simulink model "nonlin_quadro_orig"  (R2020b)
settings: Solver=VariableStepAuto  StartTime=0.0  StopTime=10.0  RelTol=1e-3
values from neighbouring files (symbols this model uses):
  b = 26.5e-6    (= 2.65e-05)    [quadro_new_ast_test.m]
  d = 0.6e-6    (= 6e-07)    [quadro_new_ast_test.m]
  g = 9.80665    [quadro_new_ast_test.m]
  Ixx = 0.1    [quadro_new_ast_test.m]
  Iyy = 0.1    [quadro_new_ast_test.m]
  Izz = 0.1    [quadro_new_ast_test.m]
  JTP = 0.005    [quadro_new_ast_test.m]
  l = 0.175    [quadro_new_ast_test.m]
  m = 1    [quadro_new_ast_test.m]
settings Model: Creator=Наташа  LastModifiedBy=Наташа

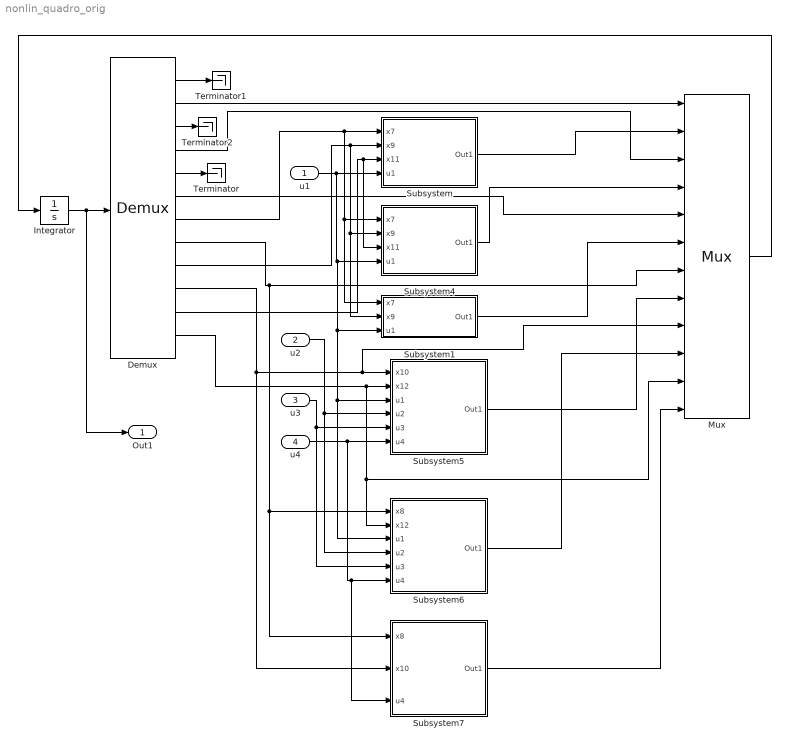
== system nonlin_quadro_orig ==
  u1 : Inport
  u2 : Inport  Port=2
  u3 : Inport  Port=3
  u4 : Inport  Port=4
  Demux : Demux  Outputs=12
  Integrator : Integrator
  Mux : Mux  Inputs=12
  Subsystem : Subsystem
  Subsystem1 : Subsystem
  Subsystem4 : Subsystem
  Subsystem5 : Subsystem
  Subsystem6 : Subsystem
  Subsystem7 : Subsystem
  Terminator : Terminator
  Terminator1 : Terminator
  Terminator2 : Terminator
  Out1 : Outport
  wires:
  Subsystem4/1(Out1) -> Mux/4
  Demux/4 -> Mux/3
  Demux/1 -> Terminator1/1
  Demux/3 -> Terminator2/1
  Demux/5 -> Terminator/1
  Subsystem6/1(Out1) -> Mux/10
  Subsystem5/1(Out1) -> Mux/8
  Demux/7 -> Subsystem1/1(x7), Subsystem4/1(x7), Subsystem/1(x7)
  u3/1 -> Subsystem6/5(u3), Subsystem5/5(u3)
  u4/1 -> Subsystem7/3(u4), Subsystem6/6(u4), Subsystem5/6(u4)
  Subsystem1/1(Out1) -> Mux/6
  u2/1 -> Subsystem6/4(u2), Subsystem5/4(u2)
  Demux/8 -> Subsystem7/1(x8), Subsystem6/1(x8), Mux/7
  Demux/9 -> Subsystem/2(x9), Subsystem1/2(x9), Subsystem4/2(x9)
  Mux/1 -> Integrator/1
  Demux/12 -> Mux/11, Subsystem6/2(x12), Subsystem5/2(x12)
  Demux/10 -> Subsystem7/2(x10), Mux/9, Subsystem5/1(x10)
  u1/1 -> Subsystem6/3(u1), Subsystem5/3(u1), Subsystem1/3(u1), Subsystem4/4(u1), Subsystem/4(u1)
  Demux/6 -> Mux/5
  Subsystem/1(Out1) -> Mux/2
  Demux/11 -> Subsystem4/3(x11), Subsystem/3(x11)
  Integrator/1 -> Out1/1, Demux/1
  Demux/2 -> Mux/1
  Subsystem7/1(Out1) -> Mux/12

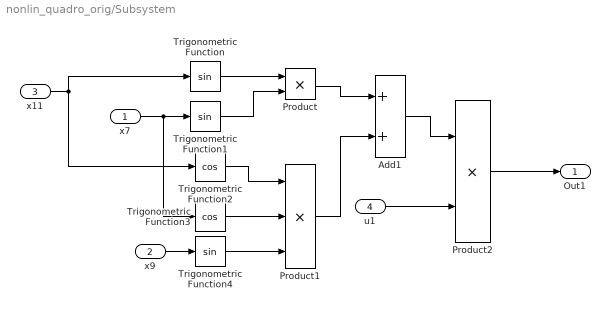
== system nonlin_quadro_orig/Subsystem ==
  x7 : Inport
  x9 : Inport  Port=2
  x11 : Inport  Port=3
  u1 : Inport  Port=4
  Add1 : Sum
  Product : Product
  Product1 : Product  Inputs=3
  Product2 : Product
  Trigonometric Function : Trigonometry
  Trigonometric Function1 : Trigonometry
  Trigonometric Function2 : Trigonometry  Operator=cos
  Trigonometric Function3 : Trigonometry  Operator=cos
  Trigonometric Function4 : Trigonometry
  Out1 : Outport
  wires:
  x11/1 -> Trigonometric Function/1, Trigonometric Function2/1
  Trigonometric Function/1 -> Product/1
  Trigonometric Function1/1 -> Product/2
  x7/1 -> Trigonometric Function3/1, Trigonometric Function1/1
  Product/1 -> Add1/1
  x9/1 -> Trigonometric Function4/1
  Trigonometric Function2/1 -> Product1/1
  Trigonometric Function3/1 -> Product1/2
  Trigonometric Function4/1 -> Product1/3
  Product1/1 -> Add1/2
  Add1/1 -> Product2/1
  u1/1 -> Product2/2
  Product2/1 -> Out1/1

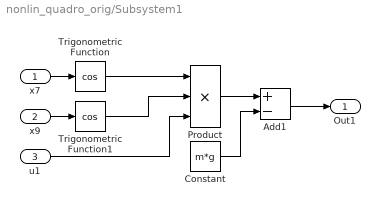
== system nonlin_quadro_orig/Subsystem1 ==
  x7 : Inport
  x9 : Inport  Port=2
  u1 : Inport  Port=3
  Add1 : Sum  Inputs=+-
  Constant : Constant  Value=m*g
  Product : Product  Inputs=3
  Trigonometric Function : Trigonometry  Operator=cos
  Trigonometric Function1 : Trigonometry  Operator=cos
  Out1 : Outport
  wires:
  x7/1 -> Trigonometric Function/1
  x9/1 -> Trigonometric Function1/1
  Trigonometric Function/1 -> Product/1
  Trigonometric Function1/1 -> Product/2
  u1/1 -> Product/3
  Product/1 -> Add1/1
  Constant/1 -> Add1/2
  Add1/1 -> Out1/1

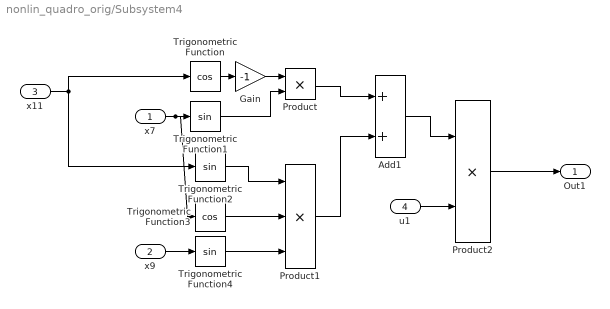
== system nonlin_quadro_orig/Subsystem4 ==
  x7 : Inport
  x9 : Inport  Port=2
  x11 : Inport  Port=3
  u1 : Inport  Port=4
  Add1 : Sum
  Gain : Gain  Gain=-1
  Product : Product
  Product1 : Product  Inputs=3
  Product2 : Product
  Trigonometric Function : Trigonometry  Operator=cos
  Trigonometric Function1 : Trigonometry
  Trigonometric Function2 : Trigonometry
  Trigonometric Function3 : Trigonometry  Operator=cos
  Trigonometric Function4 : Trigonometry
  Out1 : Outport
  wires:
  Product2/1 -> Out1/1
  u1/1 -> Product2/2
  Add1/1 -> Product2/1
  Product1/1 -> Add1/2
  Trigonometric Function4/1 -> Product1/3
  Trigonometric Function3/1 -> Product1/2
  Trigonometric Function2/1 -> Product1/1
  x9/1 -> Trigonometric Function4/1
  Product/1 -> Add1/1
  x7/1 -> Trigonometric Function3/1, Trigonometric Function1/1
  Trigonometric Function1/1 -> Product/2
  x11/1 -> Trigonometric Function2/1, Trigonometric Function/1
  Trigonometric Function/1 -> Gain/1
  Gain/1 -> Product/1

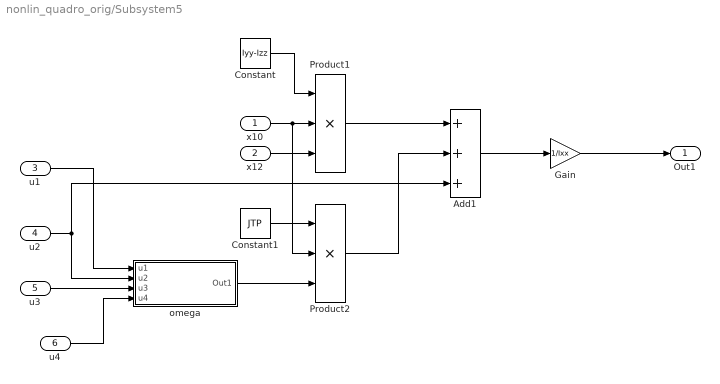
== system nonlin_quadro_orig/Subsystem5 ==
  x10 : Inport
  x12 : Inport  Port=2
  u1 : Inport  Port=3
  u2 : Inport  Port=4
  u3 : Inport  Port=5
  u4 : Inport  Port=6
  Add1 : Sum  Inputs=+++
  Constant : Constant  Value=Iyy-Izz
  Constant1 : Constant  Value=JTP
  Gain : Gain  Gain=1/Ixx
  Product1 : Product  Inputs=3
  Product2 : Product  Inputs=3
  omega : Subsystem
  Out1 : Outport
  wires:
  Constant/1 -> Product1/1
  x10/1 -> Product2/2, Product1/2
  x12/1 -> Product1/3
  Constant1/1 -> Product2/1
  omega/1(Out1) -> Product2/3
  u1/1 -> omega/1(u1)
  u2/1 -> omega/2(u2), Add1/3
  u3/1 -> omega/3(u3)
  u4/1 -> omega/4(u4)
  Product1/1 -> Add1/1
  Product2/1 -> Add1/2
  Add1/1 -> Gain/1
  Gain/1 -> Out1/1

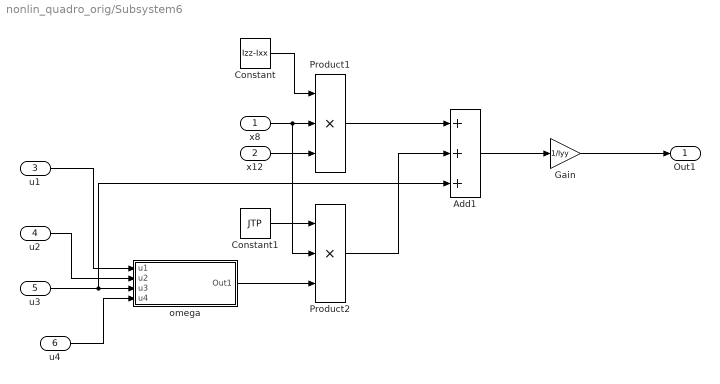
== system nonlin_quadro_orig/Subsystem6 ==
  x8 : Inport
  x12 : Inport  Port=2
  u1 : Inport  Port=3
  u2 : Inport  Port=4
  u3 : Inport  Port=5
  u4 : Inport  Port=6
  Add1 : Sum  Inputs=+++
  Constant : Constant  Value=Izz-Ixx
  Constant1 : Constant  Value=JTP
  Gain : Gain  Gain=1/Iyy
  Product1 : Product  Inputs=3
  Product2 : Product  Inputs=3
  omega : Subsystem
  Out1 : Outport
  wires:
  Gain/1 -> Out1/1
  Add1/1 -> Gain/1
  Product2/1 -> Add1/2
  Product1/1 -> Add1/1
  u4/1 -> omega/4(u4)
  u3/1 -> Add1/3, omega/3(u3)
  u2/1 -> omega/2(u2)
  u1/1 -> omega/1(u1)
  omega/1(Out1) -> Product2/3
  Constant1/1 -> Product2/1
  x12/1 -> Product1/3
  x8/1 -> Product1/2, Product2/2
  Constant/1 -> Product1/1

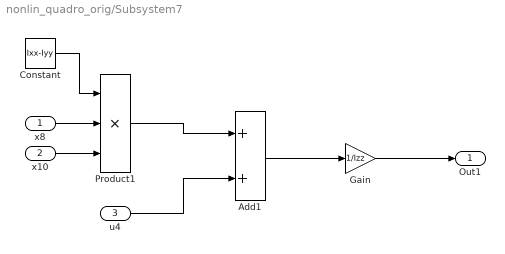
== system nonlin_quadro_orig/Subsystem7 ==
  x8 : Inport
  x10 : Inport  Port=2
  u4 : Inport  Port=3
  Add1 : Sum
  Constant : Constant  Value=Ixx-Iyy
  Gain : Gain  Gain=1/Izz
  Product1 : Product  Inputs=3
  Out1 : Outport
  wires:
  Constant/1 -> Product1/1
  x8/1 -> Product1/2
  x10/1 -> Product1/3
  Product1/1 -> Add1/1
  Add1/1 -> Gain/1
  Gain/1 -> Out1/1
  u4/1 -> Add1/2

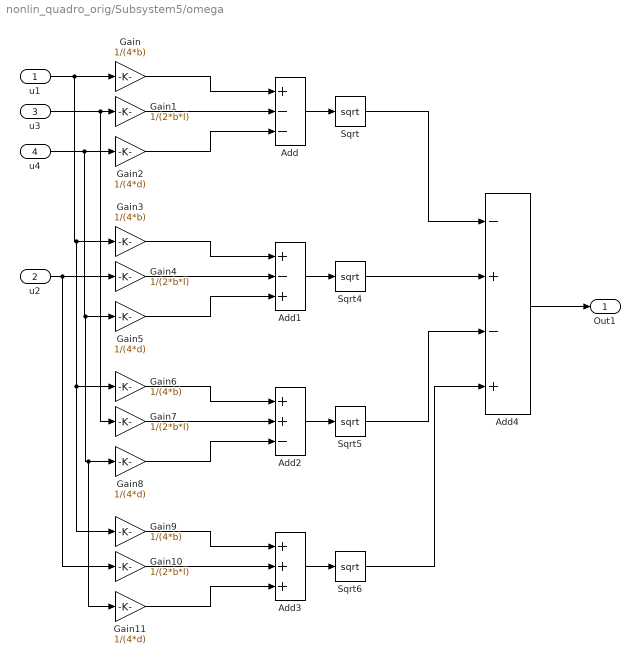
== system nonlin_quadro_orig/Subsystem5/omega ==
  u1 : Inport
  u2 : Inport  Port=2
  u3 : Inport  Port=3
  u4 : Inport  Port=4
  Add : Sum  Inputs=+--
  Add1 : Sum  Inputs=+-+
  Add2 : Sum  Inputs=++-
  Add3 : Sum  Inputs=+++
  Add4 : Sum  Inputs=-+-+
  Gain{,3,6,9} (4 alike) : Gain  Gain=1/(4*b)
  Gain{1,4,7,10} (4 alike) : Gain  Gain=1/(2*b*l)
  Gain{2,5,8,11} (4 alike) : Gain  Gain=1/(4*d)
  Sqrt{,4..6} (4 alike) : Sqrt  SaturateOnIntegerOverflow=on
  Out1 : Outport
  wires:
  Add/1 -> Sqrt/1
  u1/1 -> Gain9/1, Gain6/1, Gain3/1, Gain/1
  u3/1 -> Gain7/1, Gain1/1
  u4/1 -> Gain11/1, Gain8/1, Gain5/1, Gain2/1
  Gain2/1 -> Add/3
  Gain1/1 -> Add/2
  Gain/1 -> Add/1
  Add1/1 -> Sqrt4/1
  Gain3/1 -> Add1/1
  Gain5/1 -> Add1/3
  Gain4/1 -> Add1/2
  u2/1 -> Gain10/1, Gain4/1
  Gain8/1 -> Add2/3
  Add2/1 -> Sqrt5/1
  Gain6/1 -> Add2/1
  Gain7/1 -> Add2/2
  Gain11/1 -> Add3/3
  Add3/1 -> Sqrt6/1
  Gain9/1 -> Add3/1
  Gain10/1 -> Add3/2
  Sqrt/1 -> Add4/1
  Sqrt4/1 -> Add4/2
  Sqrt5/1 -> Add4/3
  Sqrt6/1 -> Add4/4
  Add4/1 -> Out1/1

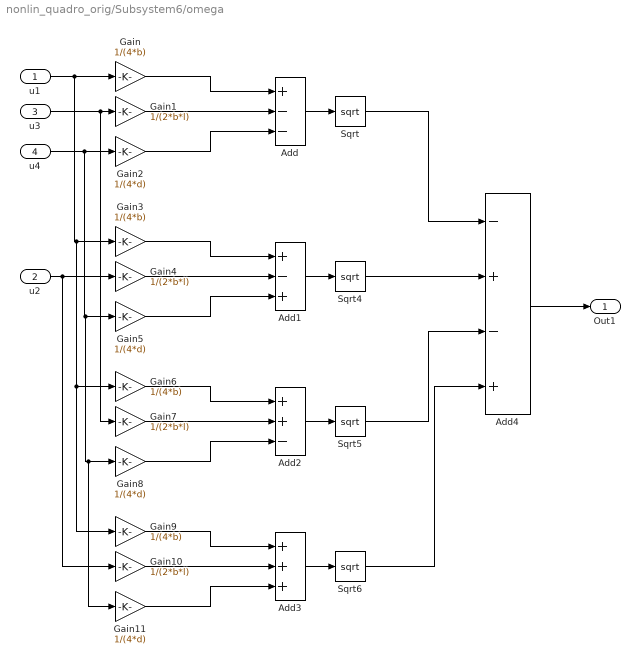
== system nonlin_quadro_orig/Subsystem6/omega ==
  u1 : Inport
  u2 : Inport  Port=2
  u3 : Inport  Port=3
  u4 : Inport  Port=4
  Add : Sum  Inputs=+--
  Add1 : Sum  Inputs=+-+
  Add2 : Sum  Inputs=++-
  Add3 : Sum  Inputs=+++
  Add4 : Sum  Inputs=-+-+
  Gain{,3,6,9} (4 alike) : Gain  Gain=1/(4*b)
  Gain{1,4,7,10} (4 alike) : Gain  Gain=1/(2*b*l)
  Gain{2,5,8,11} (4 alike) : Gain  Gain=1/(4*d)
  Sqrt{,4..6} (4 alike) : Sqrt  SaturateOnIntegerOverflow=on
  Out1 : Outport
  wires:
  Add4/1 -> Out1/1
  Sqrt6/1 -> Add4/4
  Sqrt5/1 -> Add4/3
  Sqrt4/1 -> Add4/2
  Sqrt/1 -> Add4/1
  Gain10/1 -> Add3/2
  Gain9/1 -> Add3/1
  Add3/1 -> Sqrt6/1
  Gain11/1 -> Add3/3
  Gain7/1 -> Add2/2
  Gain6/1 -> Add2/1
  Add2/1 -> Sqrt5/1
  Gain8/1 -> Add2/3
  u2/1 -> Gain4/1, Gain10/1
  Gain4/1 -> Add1/2
  Gain5/1 -> Add1/3
  Gain3/1 -> Add1/1
  Add1/1 -> Sqrt4/1
  Gain/1 -> Add/1
  Gain1/1 -> Add/2
  Gain2/1 -> Add/3
  u4/1 -> Gain2/1, Gain5/1, Gain8/1, Gain11/1
  u3/1 -> Gain1/1, Gain7/1
  u1/1 -> Gain/1, Gain3/1, Gain6/1, Gain9/1
  Add/1 -> Sqrt/1
